simulink model "Simulink_PID"  (Simulink 8.3)
settings: Solver=ode45  StartTime=0.0  StopTime=10.0  RelTol=1e-3
libraries: simulink_need_slupdate x1
settings Model: Creator=Usuario  LastModifiedBy=Lab Man
settings OptimizationCC: ExpressionDepthLimit=2147483647
settings DebuggingCC: FcnCallInpInsideContextMsg=UseLocalSettings

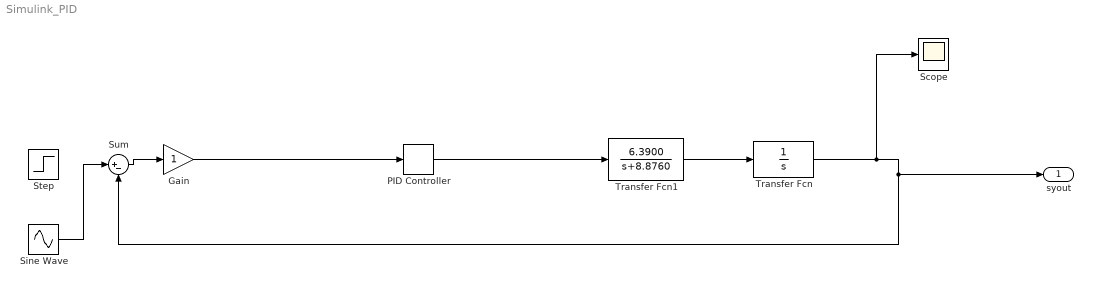
== system Simulink_PID ==
  Gain : Gain
  PID Controller : simulink_need_slupdate/PID Controller  P=7.13  I=0.0031  D=4.98
  Scope : Scope
  Sine Wave : Sin  SampleTime=0
  Step : Step  Time=0  SampleTime=0
  Sum : Sum  Inputs=|+-
  Transfer Fcn : TransferFcn  Denominator=[1 0]
  Transfer Fcn1 : TransferFcn  Numerator=[6.3900]  Denominator=[1 8.8760]
  syout : Outport
  wires:
  Transfer Fcn1/1 -> Transfer Fcn/1
  Transfer Fcn/1 -> Scope/1, Sum/2, syout/1
  Gain/1 -> PID Controller/1
  Sum/1 -> Gain/1
  PID Controller/1 -> Transfer Fcn1/1
  Sine Wave/1 -> Sum/1
